simulink model "robot_scheme"  (R2020a)
settings: Solver=ode23t  StartTime=0.0  StopTime=30  RelTol=1e-3
values from neighbouring files (symbols this model uses):
  q0 = q    [model_script.m]    (also in script_trj_q.m = [0 0 0 0 0 0]*pi/180)
settings Model: Creator=Administrator  LastModifiedBy=Administrator

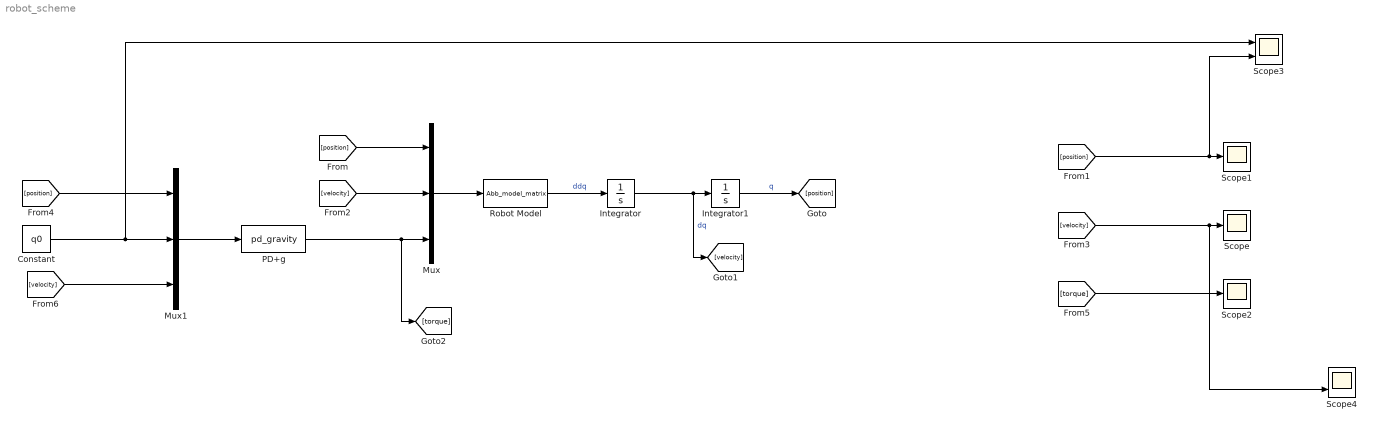
== system robot_scheme ==
  Constant : Constant  Value=q0
  Integrator : Integrator
  Integrator1 : Integrator  InitialCondition=q0
  Mux : Mux  Inputs=[6 6 6]
  Mux1 : Mux  Inputs=[6 6 6]
  PD+g : MATLABFcn  MATLABFcn=pd_gravity  OutputDimensions=6
  Robot Model : MATLABFcn  MATLABFcn=Abb_model_matrix  OutputDimensions=6
  Scope : Scope
  Scope1 : Scope
  Scope2 : Scope
  Scope3 : Scope  NumInputPorts=2
  Scope4 : Scope  NumInputPorts=2
  wires:
  Robot Model/1 -> Integrator/1  "ddq"
  Integrator/1 -> [velocity], Integrator1/1  "dq"
  Mux/1 -> Robot Model/1
  Integrator1/1 -> [position]  "q"
  [position] -> Mux/1
  [position] -> Scope3/2, Scope1/1
  [velocity] -> Mux/2
  [velocity] -> Scope4/2, Scope/1
  PD+g/1 -> [torque], Mux/3
  Mux1/1 -> PD+g/1
  [torque] -> Scope2/1
  [position] -> Mux1/1
  [velocity] -> Mux1/3
  Constant/1 -> Scope3/1, Mux1/2
